simulink model "EV_85kW_Modeling"  (R2022a)
settings: Solver=VariableStepAuto  StartTime=0  StopTime=2474  RelTol=1e-3  AbsTol=1e-3  EnableMultiTasking=on
undefined symbols (not defined in the file or in its folder): sigbuilder_block
libraries: fl_lib x18, nesl_utility x8, sdl_lib x7, ee_lib x3, autolibshared x2
settings Model: Creator=nikos  LastModifiedBy=nikos
settings SolverCC: AutoScaleAbsTol=off  ZeroCrossAlgorithm=Adaptive  AlgebraicLoopSolver=TrustRegion
settings DataIOCC: LimitDataPoints=on  MaxDataPoints=10000
settings OptimizationCC: LifeSpan=inf
settings DebuggingCC: MaskedZcDiagnostic=none  IgnoredZcDiagnostic=none  UnconnectedInputMsg=warning  UnconnectedOutputMsg=warning  UnconnectedLineMsg=warning  AllowSymbolicDim=off  PregeneratedLibrarySubsystemCodeDiagnostic=none  SFUnexpectedBacktrackingDiag=warning  SFNoUnconditionalDefaultTransitionDiag=warning  SFExecutionAtInitializationDiag=none  SFMachineParentedDataDiag=warning  ArithmeticOperatorsInVariantConditions=warning
settings SFSimCC: SimUseLocalCustomCode=off  CustomCodeUndefinedFunction=UseInterfaceOnly
settings RTWCC: RTWUseLocalCustomCode=off
settings CodeAppCC: StateflowObjectComments=on
settings GRTTargetCC: TargetLangStandard=C89/C90 (ANSI)
settings ConfigComp: CovMetricSettings=dw  CovSaveCumulativeToWorkspaceVar=on  CovSaveSingleToWorkspaceVar=on  CovExternalEMLEnable=off  CovSFcnEnable=off
settings SimscapeCC: ExplicitSolverDiagnosticOptions=none  SimscapeLogType=all  SimscapeLogDataHistory=10000

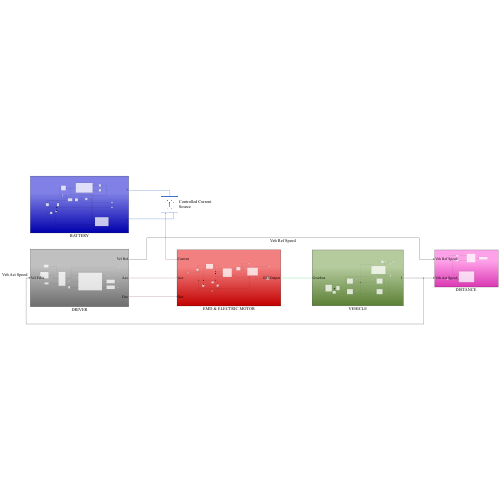
[thumbnail: Simulink's stored preview of the top-level diagram]
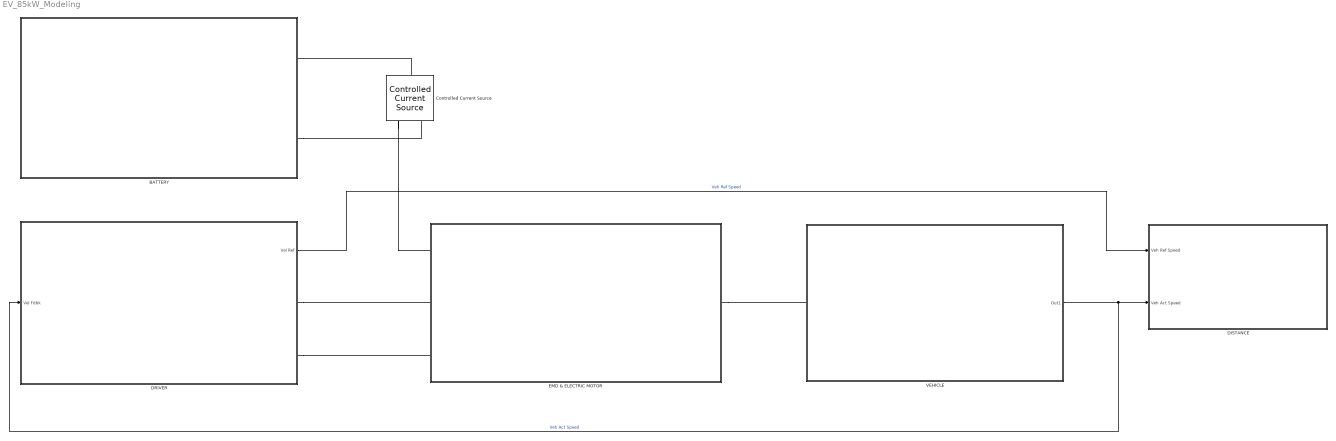
== system EV_85kW_Modeling ==
  BATTERY : Subsystem
  Controlled Current Source : fl_lib/Electrical/Electrical Sources/Controlled Current Source
      settings: SourceProductBaseCode=PW,SS,VE
  "DISTANCE " : Subsystem
  DRIVER : Subsystem
  EMD & ELECTRIC MOTOR : Subsystem
  "VEHICLE " : Subsystem
  wires:
  "VEHICLE "/1(Out1) -> DRIVER/1(Vel Fdbk), "DISTANCE "/2(Veh Act Speed)  "Veh Act Speed"
  DRIVER/1(Vel Ref) -> "DISTANCE "/1(Veh Ref Speed)  "Veh Ref Speed"
  connections:
  BATTERY/RConn2 -- Controlled Current Source/RConn2
  Controlled Current Source/LConn1 -- BATTERY/RConn1
  Controlled Current Source/RConn1 -- EMD & ELECTRIC MOTOR/RConn1
  EMD & ELECTRIC MOTOR/LConn1 -- "VEHICLE "/LConn1
  DRIVER/RConn1 -- EMD & ELECTRIC MOTOR/RConn2
  DRIVER/RConn2 -- EMD & ELECTRIC MOTOR/RConn3

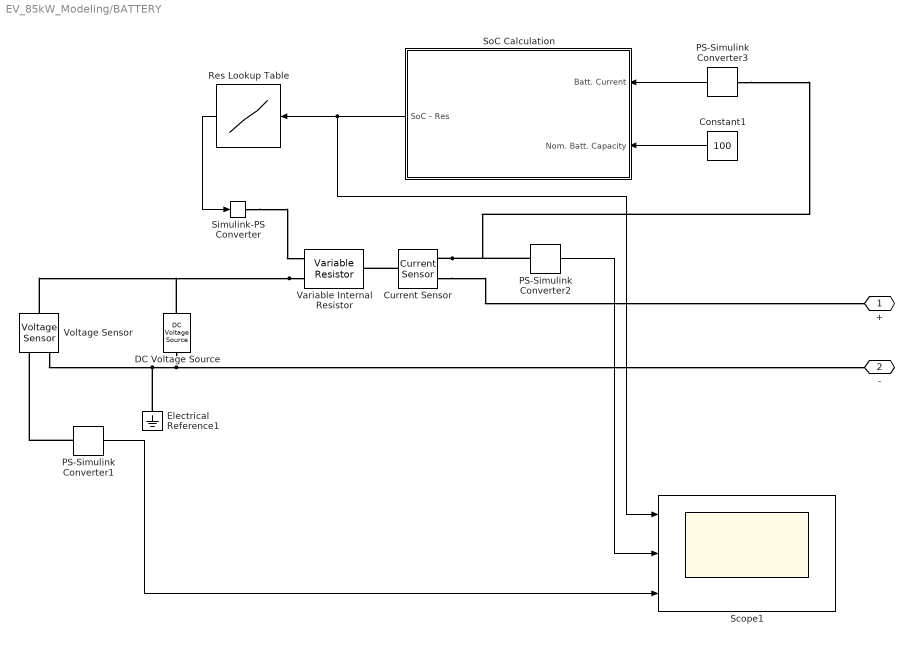
== system EV_85kW_Modeling/BATTERY ==
  Constant1 : Constant  Value=100
  Current Sensor : fl_lib/Electrical/Electrical Sensors/Current Sensor
      settings: SourceProductBaseCode=PW,SS,VE
  DC Voltage Source : fl_lib/Electrical/Electrical Sources/DC Voltage Source  v0=300 V
      settings: SourceProductBaseCode=PW,SS,VE
  Electrical Reference1 : fl_lib/Electrical/Electrical Elements/Electrical Reference
      settings: SourceProductBaseCode=PW,SS,VE
  PS-Simulink Converter1 : nesl_utility/PS-Simulink Converter  PhysicalDomain=network_engine_domain  SubClassName=ps_output  LeftPortType=input  RightPortType=output  PseudoPeriodic=off  Frequencies=[]  VectorFormat=1-D array  Unit=1  AffineConversion=off
      settings: SourceProductBaseCode=SS,PW,VE
  PS-Simulink Converter2 : nesl_utility/PS-Simulink Converter  PhysicalDomain=network_engine_domain  SubClassName=ps_output  LeftPortType=input  RightPortType=output  PseudoPeriodic=off  Frequencies=[]  VectorFormat=1-D array  Unit=1  AffineConversion=off
      settings: SourceProductBaseCode=SS,PW,VE
  PS-Simulink Converter3 : nesl_utility/PS-Simulink Converter  PhysicalDomain=network_engine_domain  SubClassName=ps_output  LeftPortType=input  RightPortType=output  PseudoPeriodic=off  Frequencies=[]  VectorFormat=1-D array  Unit=1  AffineConversion=off
      settings: SourceProductBaseCode=SS,PW,VE
  Res Lookup Table : Lookup_n-D  NumberOfTableDimensions=1  BreakpointsForDimension1=[0, 10, 20, 30, 40, 50, 60, 70, 80, 90, 100]  Table=[0.011448, 0.011038, 0.011281, 0.011236, 0.010959, 0.010714, 0.010698, 0.010712, 0.010917, 0.011304, 0.011603]  InternalRulePriority=Speed  RndMeth=Simplest
  Scope1 : Scope  NumInputPorts=3
  Simulink-PS Converter : nesl_utility/Simulink-PS Converter  PhysicalDomain=network_engine_domain  SubClassName=ps_input  LeftPortType=input  RightPortType=output  PseudoPeriodic=off  Frequencies=[]  NoiseDistribution=none  NoiseParameters=[]  Unit=1  AffineConversion=off  FilteringAndDerivatives=provide  SimscapeFilterOrder=1  InputFilterTimeConstant=0.001  UdotUserProvided=0
      settings: SourceProductBaseCode=SS,PW,VE
  SoC Calculation : Subsystem
  Variable Internal Resistor : fl_lib/Electrical/Electrical Elements/Variable Resistor  Rmin=1 Ohm  i_specify=off  i_priority=High  i=0 A  i_nominal_specify=off  i_nominal_unit=A  i_nominal_value=1  v_specify=off  v_priority=High  v=0 V  v_nominal_specify=off  v_nominal_unit=V  v_nominal_value=1
      settings: SourceProductBaseCode=PW,SS,VE
  Voltage Sensor : fl_lib/Electrical/Electrical Sensors/Voltage Sensor
      settings: SourceProductBaseCode=PW,SS,VE
  + : PMIOPort  Side=Right
  - : PMIOPort  Port=2  Side=Right
  wires:
  Constant1/1 -> SoC Calculation/2("Nom. Batt. Capacity ")
  PS-Simulink Converter1/1 -> Scope1/3
  PS-Simulink Converter3/1 -> SoC Calculation/1("Batt. Current ")
  Res Lookup Table/1 -> Simulink-PS Converter/1
  SoC Calculation/1(SoC - Res) -> Scope1/1, Res Lookup Table/1
  PS-Simulink Converter2/1 -> Scope1/2
  connections:
  Simulink-PS Converter/RConn1 -- Variable Internal Resistor/LConn1
  Current Sensor/LConn1 -- Variable Internal Resistor/RConn1
  Current Sensor/RConn1 -- PS-Simulink Converter3/LConn1 -- PS-Simulink Converter2/LConn1
  Current Sensor/RConn2 -- +/RConn1
  Variable Internal Resistor/LConn2 -- Voltage Sensor/LConn1 -- DC Voltage Source/LConn1
  Voltage Sensor/RConn2 -- Electrical Reference1/LConn1 -- -/RConn1 -- DC Voltage Source/RConn1
  PS-Simulink Converter1/LConn1 -- Voltage Sensor/RConn1

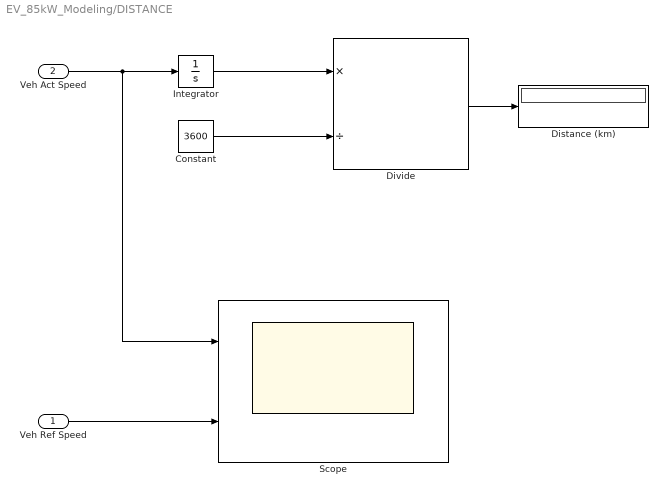
== system EV_85kW_Modeling/DISTANCE  ==
  Veh Ref Speed : Inport
  Veh Act Speed : Inport  Port=2
  Constant : Constant  Value=3600
  Distance (km) : Display
  Divide : Product  Inputs=*/
  Integrator : Integrator
  Scope : Scope  NumInputPorts=2
  wires:
  Divide/1 -> Distance (km)/1
  Constant/1 -> Divide/2
  Integrator/1 -> Divide/1
  Veh Ref Speed/1 -> Scope/2
  Veh Act Speed/1 -> Scope/1, Integrator/1

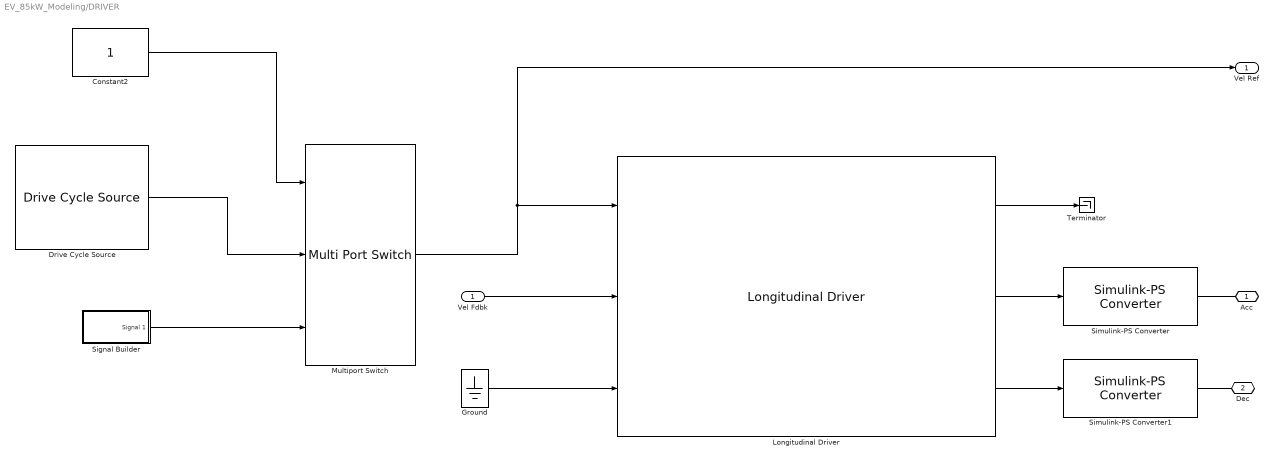
== system EV_85kW_Modeling/DRIVER ==
  Vel Fdbk : Inport
  Constant2 : Constant
  Drive Cycle Source : autolibshared/Drive Cycle Source  cycleVar=FTP75  fileVar=cycleFTP75.mat  tfinal="2474  seconds"  cycleRepeat=off  outAccPort=off  outGearPort=off  gearList=No gear data  t_wot1=5  xdot_woto=0  xdot_wot1=30  t_wot2=20  xdot_wot2=0  t_wotend=30  srcUnit=m/s  outUnit=m/s  srcAccUnit=m/s/s  outAccUnit=m/s^2  dt=0  aMode=1  faultOption=off  velBnd=2  velBndUnit=mph  inUnit=m/s  timeBnd=1  failOption=off  stopSim=off  maxFaultCnt=10  maxFaultTime=2  maxTotFaultTime=15  traceOption=off  dtTrace=1  traceWindow=10  lastDCname=FTP75  lastOutUnit=mph  lastDT=0  lastTB=1  lastSB=2  forceCalcBound=off
      settings: SourceProductBaseCode=PW,DR,MT,VE
  Ground : Ground
  Longitudinal Driver : autolibshared/Longitudinal Driver  extAccelOvr=off  extDecelOvr=off  extAccelHld=off  extDecelHld=off  extAccelZero=off  extDecelZero=off  cntrlType=PI  shftType=None  velUnits=km/h  gearOut=off  Kp=10  Ki=5  Kff=.1  Kg=0  VehVelVec=[0 100]  KffVec=[.1 .1]  KpVec=[10 10]  KiVec=[5 5]  KgVec=[0 0]  m=1500  Kpt=3000  tau=.1  L=2  aR=200  bR=2.5  cR=.5  g=9.81  vnom=5  Kaw=1  tauerr=.01  tauPt=2  GearInit=0  tShift=.1  pdlVec=[0.1 0.4 0.5 0.9]  upShftTbl=[-1 12.9375 26.4375 39.9375 51.18749999999999 62.4375 72.84375 83.25;-1 16.3125 29.8125 43.3125 54.5624 65.8125 76.78125 87.75;-1 19.6875 33.1875 46.68749999999999 57.9375 69.1875 80.71875 92.25;-1 33 52.5 77.25 100.5 138.75 161.875 185]  dwnShftTbl=[1 9.5625 23.0625 36.5625 47.8125 59.0625 68.90625 78.75;1 12.9375 26.4375 39.9375 51.18749999999999 62.4375 72.84375 83.25;1 16.3125 29.8125 43.3125 54.562499 65.8125 76.78125 87.75;1 19.6875 33.1875 46.68749999999999 57.9375 69.1875 80.71875 92.25]  tClutch=.5  tRev=.5  tPark=120  aMode=2  UpGearVec="[0  1  2  3  4  5  6  7]"  DownGearVec="[1  2  3  4  5  6  7  8]"
      settings: SourceProductBaseCode=PW,DR,MT,VE
  Multiport Switch : MultiPortSwitch  Inputs=2  SaturateOnIntegerOverflow=off  InputSameDT=off
  Signal Builder : Subsystem  Tag=STV Subsys  LoadFcn=sigbuilder_block('load');  StartFcn=sigbuilder_block('start');  StopFcn=sigbuilder_block('stop');  ClipboardFcn=sigbuilder_block('clipboard');  mask(Sigbuilder block){tuvar=[0:10]}
      mask help: Simulink:masks:SigbuilderBlock_MD
      mask init:
      | if ~strcmp(get_param(bdroot(gcbh),'SimulationStatus'),'stopped') tuvar = sigbuilder_block('maskInit'); end
      settings: CopyFcn=sigbuilder_block('copy');  DeleteFcn=sigbuilder_block('delete');  ModelCloseFcn=sigbuilder_block('modelClose');  PreSaveFcn=sigbuilder_block('preSave');  PauseFcn=sigbuilder_block('pause');  ContinueFcn=sigbuilder_block('continue');  NameChangeFcn=sigbuilder_block('namechange');  OpenFcn=sigbuilder_block('open',[0 30 1152 561.6 ]);  CloseFcn=sigbuilder_block('close');
      mask Display: plot(0, 0, 100, 100,[2, 2, 32, 32, 2], [68, 8, 8, 68, 68],[32, 2], [38, 38], [32, 19, 2],[53, 60, 44], [32, 17, 17, 2],[16, 16, 31, 31]);txt = getActiveGroup(gcbh);text(2, 100, txt,'verticalAlignment', 'top');
  Simulink-PS Converter : nesl_utility/Simulink-PS Converter  PhysicalDomain=network_engine_domain  SubClassName=ps_input  LeftPortType=input  RightPortType=output  PseudoPeriodic=off  Frequencies=[]  NoiseDistribution=none  NoiseParameters=[]  Unit=1  AffineConversion=off  FilteringAndDerivatives=provide  SimscapeFilterOrder=1  InputFilterTimeConstant=0.001  UdotUserProvided=0
      settings: SourceProductBaseCode=SS,PW,VE
  Simulink-PS Converter1 : nesl_utility/Simulink-PS Converter  PhysicalDomain=network_engine_domain  SubClassName=ps_input  LeftPortType=input  RightPortType=output  PseudoPeriodic=off  Frequencies=[]  NoiseDistribution=none  NoiseParameters=[]  Unit=1  AffineConversion=off  FilteringAndDerivatives=provide  SimscapeFilterOrder=1  InputFilterTimeConstant=0.001  UdotUserProvided=0
      settings: SourceProductBaseCode=SS,PW,VE
  Terminator : Terminator
  Acc : PMIOPort  Side=Right
  Dec : PMIOPort  Port=2  Side=Right
  Vel Ref : Outport  VectorParamsAs1DForOutWhenUnconnected=off
  wires:
  Vel Fdbk/1 -> Longitudinal Driver/2
  Longitudinal Driver/2 -> Simulink-PS Converter/1
  Ground/1 -> Longitudinal Driver/3
  Longitudinal Driver/3 -> Simulink-PS Converter1/1
  Drive Cycle Source/1 -> Multiport Switch/2
  Constant2/1 -> Multiport Switch/1
  Multiport Switch/1 -> Vel Ref/1, Longitudinal Driver/1
  Signal Builder/1(Signal 1) -> Multiport Switch/3
  Longitudinal Driver/1 -> Terminator/1
  connections:
  Simulink-PS Converter/RConn1 -- Acc/RConn1
  Simulink-PS Converter1/RConn1 -- Dec/RConn1

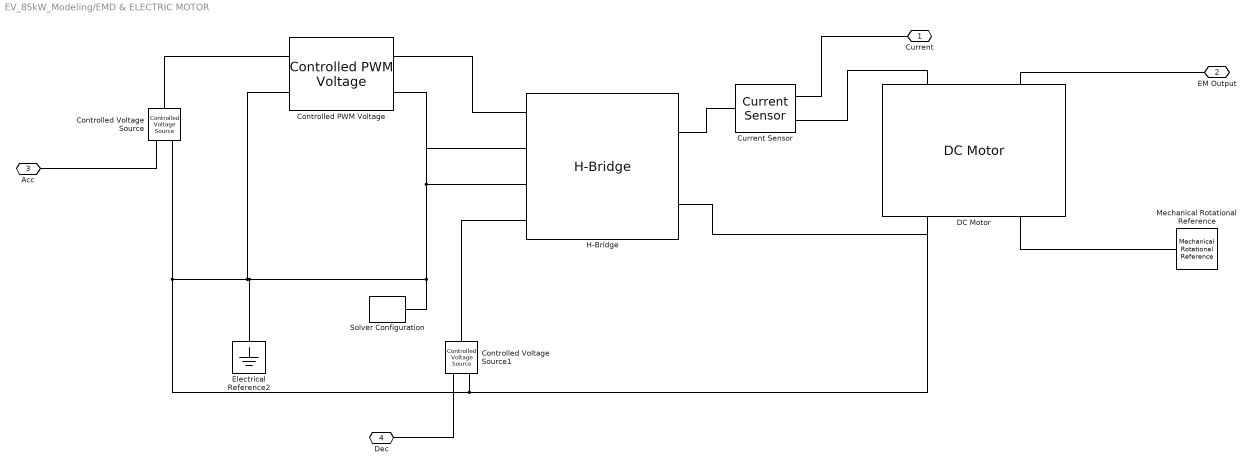
== system EV_85kW_Modeling/EMD & ELECTRIC MOTOR ==
  Controlled PWM Voltage : ee_lib/Integrated Circuits/Controlled PWM Voltage  F=4000 Hz  TD=0 s  pulse_width_offset=0 s  pulse_min=0 s  pwm_or_av=2  event_type=1  sample_time=1e-6 s  Vmin=0 V  Vmax=1 V  Vm=5 V  u_min=0  u_max=1
  Controlled Voltage Source : fl_lib/Electrical/Electrical Sources/Controlled Voltage Source
      settings: SourceProductBaseCode=PW,SS,VE
  Controlled Voltage Source1 : fl_lib/Electrical/Electrical Sources/Controlled Voltage Source
      settings: SourceProductBaseCode=PW,SS,VE
  Current Sensor : fl_lib/Electrical/Electrical Sensors/Current Sensor
      settings: SourceProductBaseCode=PW,SS,VE
  DC Motor : ee_lib/Electromechanical/Brushed Motors/DC Motor  field_option=ee.enum.field_option.pm  Rf=100 Ohm  Lf=1 H  Laf=0.15 H  If0=0 A  parameterization=ee.enum.dcparam_option.load_speed  Ra=3.9 Ohm  La=12e-6 H  emf_or_torque=ee.enum.emf_or_torque.kv  Kv=0.072e-3 V/rpm  Ki=6.876e-4 N*m/A  T_stall=0.24e-3 N*m  w_max=10000 rpm  w_rated=3796 rpm  P_rated=150 kW  V_rated=300 V  lam_param=ee.enum.lam_param.damping  i_noload=0 A  V_i_noload=1.5 V  J=0.01 cm^2*g  lam=0 N*m*s/rad  speed0=0 rpm  enable_fault_armature=simscape.enum.onoff.off  rev_faulted=1 / 3  G_faulted_armature=1e-5 S  fault_trigger_armature=ee.enum.faults.faultTrigger.temporal  t_fault_armature=1 s  max_permissible_current_armature=inf A  t_fail_on_current_armature=1 s  enable_fault_field=simscape.enum.onoff.off  G_faulted_field=1e-5 S  fault_trigger_field=ee.enum.faults.faultTrigger.temporal  t_fault_field=1 s  max_permissible_current_field=inf A  t_fail_on_current_field=1 s  fault_action=simscape.enum.assert.action.none  alpha=3.93e-3 1/K  Tmeas=25 degC  thermal_mass=100 J/K  initial_temperature=25 degC
  Electrical Reference2 : fl_lib/Electrical/Electrical Elements/Electrical Reference
      settings: SourceProductBaseCode=PW,SS,VE
  H-Bridge : ee_lib/Semiconductors & Converters/Converters/H-Bridge  supply_ports=ee.enum.supply_ports.hidesupply  pwm_or_av=ee.enum.pwm_or_av.averaged  regenerative_braking_mode=ee.enum.converters.regenerative_braking_mode.always_enabled  discontinuous=0  freewheeling_mode=3  Rload=10 Ohm  Lload=1e-5 H  F=10 kHz  Venable=2.5 V  Vmax=5.0 V  Vreverse=2.5 V  Vbrake=2.5 V  Vm=300 V  Ron=0.1 Ohm  Don=0.05 Ohm  Goff=1e-6 S  Tmeas=298.15 K  Ron2=0.1 Ohm  Don2=0.05 Ohm  Tmeas2=398.15 K  thermal_mass=100 J/K  initial_temperature=298.15 K
  Mechanical Rotational Reference : fl_lib/Mechanical/Rotational Elements/Mechanical Rotational Reference
      settings: SourceProductBaseCode=PW,SS,VE
  Solver Configuration : nesl_utility/Solver Configuration  PhysicalDomain=network_engine_domain  SubClassName=solver  LeftPortType=input  RightPortType=generic  Tones=[]  Harmonics=[]  SimulateNoise=off  Profile=off  UseLocalSampling=off  EnableSwitchedLinearOptims=on  FrequencyDomain=off  UseCCode=off  RelTol=0.001  AbsTol=0.001  MinStep=1e-09  ToWorkspace=off  RevertToSquareIcSolve=off  NumHomotopyIterations=100  PhasorMode=off  PhasorModeNumHarmonics=1  IndexReductionMethod=DerivativeReplacement  DoDC=off  ResidualTolerance=1e-09  UseLocalSolver=off  LocalSolverChoice=NE_BACKWARD_EULER_ADVANCER  LocalSolverSampleTime=0.001  DoFixedCost=off  MaxNonlinIter=3  MaxModeIter=2  ComputeImpulses=off  ImpulseIterations=2  LinearAlgebra=auto  LinearAlgebraNumThread=0  EquationFormulation=NE_TIME_EF  DelaysMemoryBudget=1024  AutomaticFiltering=on  FilteringTimeConstant=0.001  PartitionStorageMethod=AS_NEEDED  PartitionMemoryBudget=1024  PartitionMethod=ROBUST
      settings: SourceProductBaseCode=SS,PW,VE
  Current : PMIOPort  Side=Right
  EM Output : PMIOPort  Port=2  Side=Left
  Acc : PMIOPort  Port=3  Side=Right
  Dec : PMIOPort  Port=4  Side=Right
  connections:
  Mechanical Rotational Reference/LConn1 -- DC Motor/RConn2
  DC Motor/RConn1 -- H-Bridge/RConn2 -- Controlled Voltage Source/RConn2 -- Solver Configuration/RConn1 -- H-Bridge/LConn3 -- Controlled PWM Voltage/RConn2 -- H-Bridge/LConn2 -- Electrical Reference2/LConn1 -- Controlled PWM Voltage/LConn2 -- Controlled Voltage Source1/RConn2
  H-Bridge/LConn4 -- Controlled Voltage Source1/LConn1
  Controlled Voltage Source/LConn1 -- Controlled PWM Voltage/LConn1
  DC Motor/LConn1 -- Current Sensor/RConn2
  DC Motor/LConn2 -- EM Output/RConn1
  Current Sensor/LConn1 -- H-Bridge/RConn1
  H-Bridge/LConn1 -- Controlled PWM Voltage/RConn1
  Current/RConn1 -- Current Sensor/RConn1
  Acc/RConn1 -- Controlled Voltage Source/RConn1
  Dec/RConn1 -- Controlled Voltage Source1/RConn1

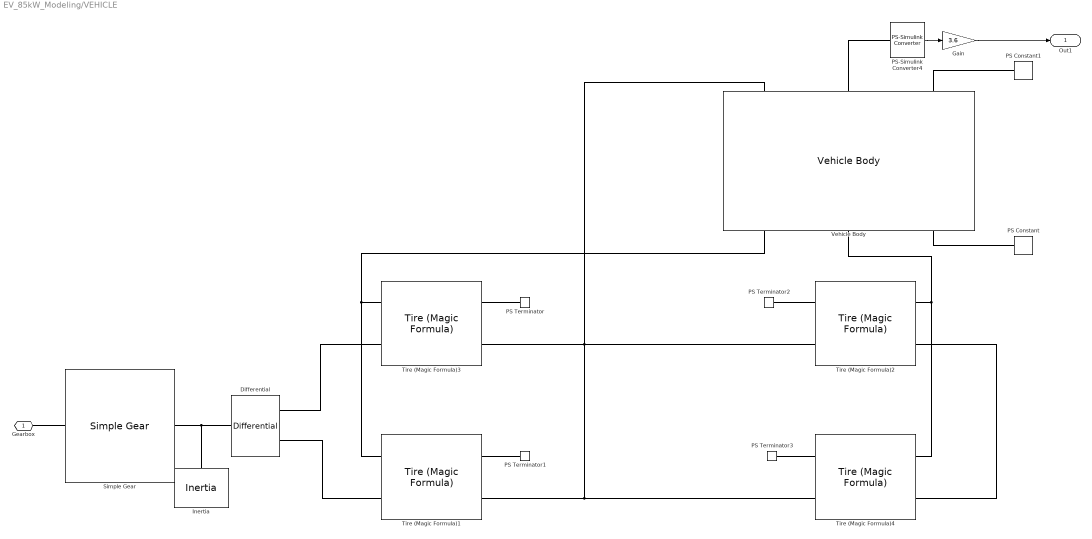
== system EV_85kW_Modeling/VEHICLE  ==
  Differential : sdl_lib/Gears/Differential  driveshaft_location=2  cd_ratio=4  friction_model=1  efficiency=[.85, .92]  temperature_TLU=[280, 300, 320] K  efficiency_ss_TLU=[.95, .9, .85]  efficiency_cd_TLU=[.95, .9, .85]  pwr_thr=[.001, .001] W  mu_visc=[0, 0] N*m/(rad/s)  model_inertia=0  carrier_inertia=0.001 kg*m^2  planet_inertia=0.001 kg*m^2  thermal_mass=50 J/K  T_init=300 K
      settings: SourceProductBaseCode=LD
  Gain : Gain  Gain=3.6
  Inertia : fl_lib/Mechanical/Rotational Elements/Inertia  inertia=0.01 kg*m^2  num_ports=foundation.enum.numPorts2.one  w_specify=off  w_priority=High  w=0 rad/s  w_nominal_specify=off  w_nominal_unit=rad/s  w_nominal_value=1  t_specify=off  t_priority=None  t=0 N*m  t_nominal_specify=off  t_nominal_unit=N*m  t_nominal_value=1
      settings: SourceProductBaseCode=PW,SS,VE
  PS Constant : fl_lib/Physical Signals/Sources/PS Constant  constant=0
      settings: SourceProductBaseCode=PW,SS,VE
  PS Constant1 : fl_lib/Physical Signals/Sources/PS Constant  constant=0
      settings: SourceProductBaseCode=PW,SS,VE
  PS Terminator{,1..3} (4 alike) : fl_lib/Physical Signals/Sinks/PS Terminator
      settings: SourceProductBaseCode=PW,SS,VE
  PS-Simulink Converter4 : nesl_utility/PS-Simulink Converter  PhysicalDomain=network_engine_domain  SubClassName=ps_output  LeftPortType=input  RightPortType=output  PseudoPeriodic=off  Frequencies=[]  VectorFormat=inherit  Unit=1  AffineConversion=off
      settings: SourceProductBaseCode=SS,PW,VE
  Simple Gear : sdl_lib/Gears/Simple Gear  ratio=6  rotation_direction=sdl.enum.shaftOutputDirection.same  friction_model=sdl.enum.gear_efficiencies_load.off  T_noload=0.1 N*m  T_nom=5 N*m  efficiency_nom=0.8  efficiency=0.8  temperature_TLU=[ 280 300 320 ] K  load_TLU=[ 1 5 10 ] N*m  efficiency_TLU=[ 0.95 0.9 0.85 ]  efficiency_TLU2=[ 0.85 0.8 0.75; 0.95 0.9 0.85; 0.85 0.8 0.7 ]  w_thr=0.01 rad/s  pwr_thr=0.001 W  backlash_model=sdl.enum.backlashModel.Off  backlash_distance=1e-3 mm  x0=0 mm  r_base=0.1 m  hardstop_model=simscape.enum.hardstop.smooth  transition=1e-4 mm  backlash_stiffness=1e7 N/m  backlash_damping=1e6 N*s/m  e=0  v_tol=0.001 m/s  mu_visc=[ 0 0 ] N*m/(rad/s)  enable_faults=simscape.enum.onoff.off  efficiency_fault=0.05  external_fault=simscape.enum.onoff.off  temporal_fault=simscape.enum.onoff.off  fault_time=5 s  fault_angles=pi / 12 rad  report_fault=(1)-1  thermal_mass=50 J/K  temperature_specify=off  temperature_priority=High  temperature=300 K  temperature_nominal_specify=off  temperature_nominal_unit=K  temperature_nominal_value=1  x_backlash_specify=off  x_backlash_priority=None  x_backlash=0 mm  x_backlash_nominal_specify=off  x_backlash_nominal_unit=mm  x_backlash_nominal_value=1  f_hardstop_specify=off  f_hardstop_priority=None  f_hardstop=0 N  f_hardstop_nominal_specify=off  f_hardstop_nominal_unit=N  f_hardstop_nominal_value=1  v_backlash_specify=off  v_backlash_priority=None  v_backlash=0 m/s  v_backlash_nominal_specify=off  v_backlash_nominal_unit=m/s  v_backlash_nominal_value=1
  Tire (Magic Formula){1..4} (4 alike) : sdl_lib/Tires & Vehicles/Tire (Magic Formula)  parameterization=sdl.enum.magic_tire_model.load  F_z1=3e+3 N  F_x1=3.5e+3 N  kappa1=10  B_m=10  C_m=1.9  D_m=1  E_m=0.97  fz0=3500 N  p_Cx=1.685  p_Dx=[ 1.21 -0.037 ]  p_Ex=[ 0.344 0.095 -0.02 0 ]  p_Kx=[ 21.51 -0.163 0.245 ]  p_Hx=[ -0.002 0.002 ]  p_Vx=[ 0 0 ]  r_e=0.3 m  model_compliance=0  stiffness=1e+6 N/m  damping=1000 N/(m/s)  model_inertia=sdl.enum.model_inertia.on  inertia=1 kg*m^2  initial_velocity=0 rad/s  model_resistance=simscape.enum.onoff.on  resistance_model=1  coeff=0.022  p_tire=250e3 Pa  alpha=-0.003  beta=0.97  coeff_a=84e-4  coeff_b=6.2e-4 s/m  coeff_c=1.6e-4 s^2/m^2  v_thr=1e-3 m/s  v_tr_thr=0.1 m/s
  Vehicle Body : sdl_lib/Tires & Vehicles/Vehicle Body  mass=1470 kg  n_w=2  x_f=1.4 m  x_r=1.6 m  y_c=0.5 m  mass_var=simscape.enum.onoff.off  g=9.81 m/s^2  liftoff_warning=simscape.enum.onoff.off  area=2.91 m^2  Cd=0.15  rho=1.22 kg/m^3  model_pitch=simscape.enum.onoff.off  inertia=4000 kg*m^2  suspension_model=sdl.enum.linearTLU.linear  k_f=1e4 N/m  b_f=1e4 N/(m/s)  k_r=1e4 N/m  b_r=1e4 N/(m/s)  k_f_TLU=[-2000, -1000, 0, 1000, 2000] N  x_f_TLU=[-.4, -.2, 0, .2, .4] m  b_f_TLU=[-200, -100, 0, 100, 200] N  v_f_TLU=[-4, -2, 0, 2, 4] m/s  k_r_TLU=[-2000, -1000, 0, 1000, 2000] N  x_r_TLU=[-.4, -.2, 0, .2, .4] m  b_r_TLU=[-200, -100, 0, 100, 200] N  v_r_TLU=[-4, -2, 0, 2, 4] m/s  interp_method=simscape.enum.interpolation.linear  extrap_method=simscape.enum.extrapolation.linear  model_hardstop=simscape.enum.onoff.off  upper_bound_f=.25 m  lower_bound_f=-.25 m  stop_k_f=1e6 N/m  stop_b_f=150 N/(m/s)  upper_bound_r=.25 m  lower_bound_r=-.25 m  stop_k_r=1e6 N/m  stop_b_r=150 N/(m/s)  initial_pitch=0 rad  initial_pitch_rate=0 rad/s  v_specify=on  v_priority=High  v=0 m/s  v_nominal_specify=off  v_nominal_unit=m/s  v_nominal_value=1
  Gearbox : PMIOPort  Side=Left
  Out1 : Outport  VectorParamsAs1DForOutWhenUnconnected=off
  wires:
  PS-Simulink Converter4/1 -> Gain/1
  Gain/1 -> Out1/1
  connections:
  Vehicle Body/LConn1 -- Tire (Magic Formula)2/RConn2 -- Tire (Magic Formula)4/RConn2 -- Tire (Magic Formula)1/RConn2 -- Tire (Magic Formula)3/RConn2
  Tire (Magic Formula)4/LConn2 -- Tire (Magic Formula)2/LConn2
  Tire (Magic Formula)1/RConn1 -- PS Terminator1/LConn1
  Gearbox/RConn1 -- Simple Gear/LConn1
  Vehicle Body/RConn2 -- Tire (Magic Formula)4/LConn1 -- Tire (Magic Formula)2/LConn1
  Tire (Magic Formula)3/LConn1 -- Tire (Magic Formula)1/LConn1 -- Vehicle Body/RConn1
  PS Terminator/LConn1 -- Tire (Magic Formula)3/RConn1
  Tire (Magic Formula)1/LConn2 -- Differential/RConn1
  PS-Simulink Converter4/LConn1 -- Vehicle Body/LConn2
  Differential/LConn1 -- Inertia/LConn1 -- Simple Gear/RConn1
  Tire (Magic Formula)2/RConn1 -- PS Terminator2/LConn1
  Tire (Magic Formula)4/RConn1 -- PS Terminator3/LConn1
  Differential/RConn2 -- Tire (Magic Formula)3/LConn2
  PS Constant/RConn1 -- Vehicle Body/RConn3
  PS Constant1/RConn1 -- Vehicle Body/LConn3

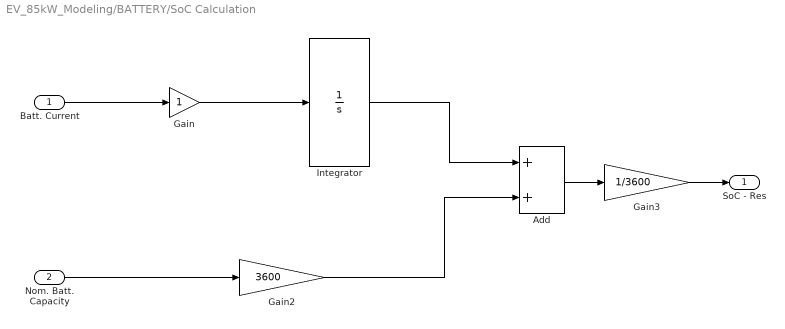
== system EV_85kW_Modeling/BATTERY/SoC Calculation ==
  "Batt. Current " : Inport
  "Nom. Batt. Capacity " : Inport  Port=2  OutMin=0  OutMax=100
  Add : Sum
  Gain : Gain
  Gain2 : Gain  Gain=3600
  Gain3 : Gain  Gain=1/3600
  Integrator : Integrator
  SoC - Res : Outport  VectorParamsAs1DForOutWhenUnconnected=off
  wires:
  "Batt. Current "/1 -> Gain/1
  Gain/1 -> Integrator/1
  "Nom. Batt. Capacity "/1 -> Gain2/1
  Gain2/1 -> Add/2
  Add/1 -> Gain3/1
  Integrator/1 -> Add/1
  Gain3/1 -> SoC - Res/1

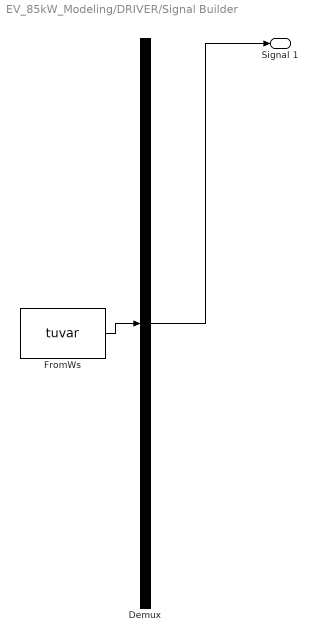
== system EV_85kW_Modeling/DRIVER/Signal Builder ==
  Demux : Demux  Tag=STV Demux  Outputs=1
      settings: DisplayOption=none
  FromWs : FromWorkspace  Tag=STV FromWs  VariableName=tuvar
      SigBuilderData=|
      | common.afterFinalStr = 'Extrapolate'
      | common.sampleTime = 0
      | dataSet.timeRange = [0 10]
      | dataSet.name = 'Group 1'
      | sbobj.Groups.Name = 'Group 1'
      | sbobj.Groups.Signals.Name = 'Signal 1'
      | sbobj.Groups.Signals.XData = [0 0.76 0.76 4.87 4.87 10]
      | sbobj.Groups.Signals.YData = [0 0 1.8 85.6 -24.2 0]
  Signal 1 : Outport  Tag=STV Outport
  wires:
  Demux/1 -> Signal 1/1
  FromWs/1 -> Demux/1
